simulink model "Accel_Model"  (R2024a)
settings: Solver=FixedStepAuto  StartTime=0.0  StopTime=360  RelTol=1e-3
values from neighbouring files (symbols this model uses):
  aXbias = mean(accelX)    [parse_testing_data.m]
  aYbias = mean(accelY)    [parse_testing_data.m]
  aZbias = mean(accelZ)    [parse_testing_data.m]
libraries: aerolibnav x1
settings Model: Creator=gryet  LastModifiedBy=gryet

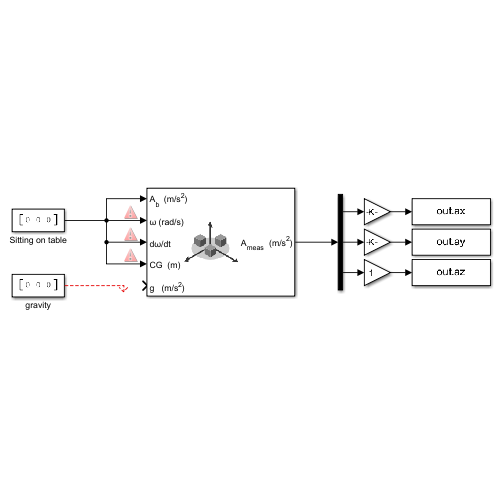
[thumbnail: Simulink's stored preview of the top-level diagram]
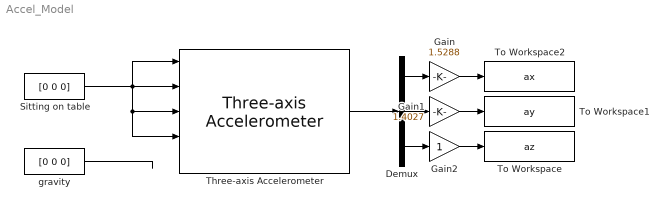
== system Accel_Model ==
  Demux : Demux  Outputs=3
  Gain : Gain  Gain=1.5288
  Gain1 : Gain  Gain=1.4027
  Gain2 : Gain
  Sitting on table : Constant  Value=[0 0 0]
  Three-axis Accelerometer : aerolibnav/Three-axis Accelerometer  units=Metric (MKS)  acc=[0 0 0]  gtype=on  dtype_a=on  w_a=190  z_a=0.707  a_sf_cc=[1 0 0; 0 1 0; 0 0 1]  a_bias=[aXbias/1.5288 aYbias/1.4027 aZbias]  a_Ts=0.0625  a_rand=on  a_seeds=[23093 23094 23095]  a_pow="[1.974e-05  1.974e-05 1.974e-05]"  a_sat="[-inf  -inf  -inf  inf inf inf]"
  To Workspace : ToWorkspace  VariableName=az  SampleTime=-1
  To Workspace1 : ToWorkspace  VariableName=ay  SampleTime=-1
  To Workspace2 : ToWorkspace  VariableName=ax  SampleTime=-1
  gravity : Constant  Value=[0 0 0]
  wires:
  Sitting on table/1 -> Three-axis Accelerometer/1, Three-axis Accelerometer/4, Three-axis Accelerometer/3, Three-axis Accelerometer/2
  gravity/1 -> ?
  Three-axis Accelerometer/1 -> Demux/1
  Demux/3 -> Gain2/1
  Demux/2 -> Gain1/1
  Demux/1 -> Gain/1
  Gain/1 -> To Workspace2/1
  Gain1/1 -> To Workspace1/1
  Gain2/1 -> To Workspace/1
